simulink model "Eight_Stator_Resistance_Speed_ctrl_of_IM"  (R2024a)
settings: Solver=ode23tb  StartTime=0.0  StopTime=10.0  MaxStep=1e-4  RelTol=1e-3
libraries: spsACVoltageSourceLib x3, spsBreakerLib x3, spsSeriesRLCBranchLib x3, spsAsynchronousMachineSIUnitsLib x1, sps_lib x1
settings Model: Creator=91889  LastModifiedBy=91889
settings DataIOCC: InitialState=[0 0 0 0 0 0 0]  LoadInitialState=on

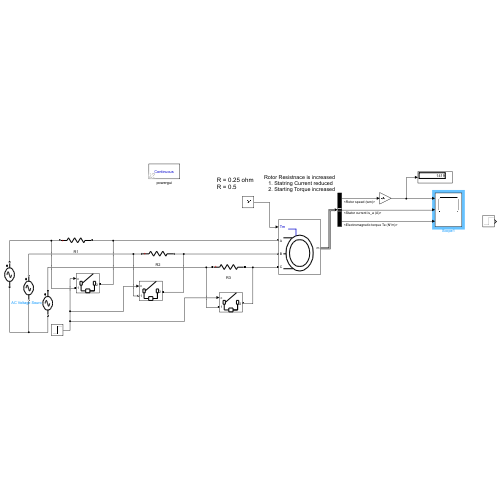
[thumbnail: Simulink's stored preview of the top-level diagram]
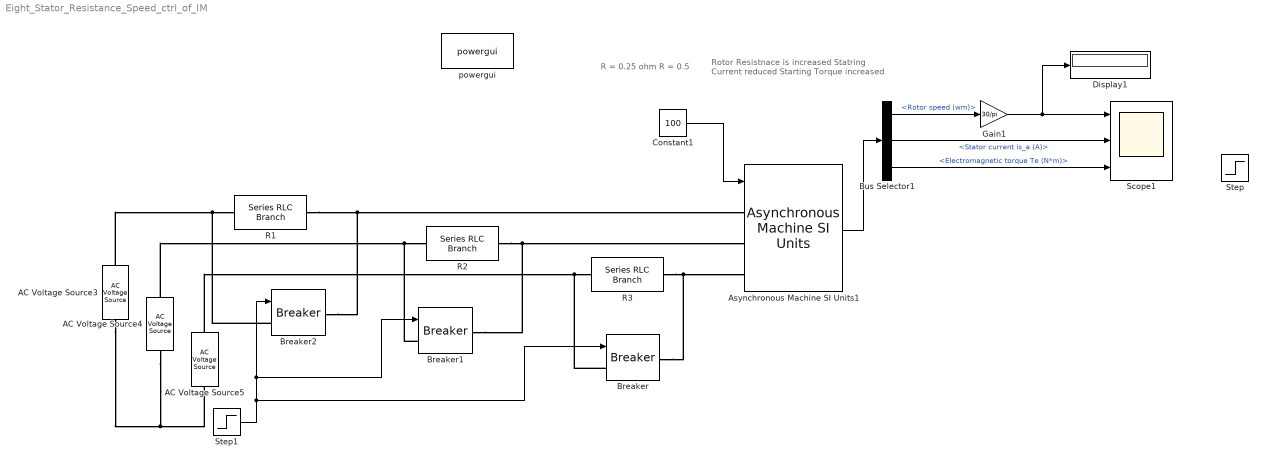
== system Eight_Stator_Resistance_Speed_ctrl_of_IM ==
  note: R = 0.25 ohm
      | R = 0.5
  note: Rotor Resistnace is increased
      | Statring Current reduced
      | Starting Torque increased
  AC Voltage Source3 : spsACVoltageSourceLib/AC Voltage Source  Amplitude=376  Phase=0  Frequency=50  SampleTime=0  Measurements=None  BusType=swing  Pref=10e3  Qref=0  Qmin=-inf  Qmax=+inf
  AC Voltage Source4 : spsACVoltageSourceLib/AC Voltage Source  Amplitude=376  Phase=-120  Frequency=50  SampleTime=0  Measurements=None  BusType=swing  Pref=10e3  Qref=0  Qmin=-inf  Qmax=+inf
  AC Voltage Source5 : spsACVoltageSourceLib/AC Voltage Source  Amplitude=376  Phase=120  Frequency=50  SampleTime=0  Measurements=None  BusType=swing  Pref=10e3  Qref=0  Qmin=-inf  Qmax=+inf
  Asynchronous Machine SI Units1 : spsAsynchronousMachineSIUnitsLib/Asynchronous Machine SI Units  RotorType=Squirrel-cage  PresetModel=No  MechanicalLoad=Torque Tm  ShowDetailedParameters=on  ReferenceFrame=Rotor  Units=SI  MeasurementBus=off  NominalParameters=[1.845e+04 400 50]  VoltageRatio=1  Stator=[0.5968 0.0003495]  Rotor=[0.6258 0.005473]  Cage1=[0.4155 0.002066]  Cage2=[0.4168 0.0003495]  Lm=0.0354  Mechanical=[0.05 0.005879 2]  PolePairs=2  InitialConditions=[0 0 0 0 0 0 0 0]  SimulateSaturation=off  Saturation=[14.03593122, 27.81365428, 53.79336849, 72.68890987, 97.98006896, 148.6815601, 215.7428561, 302.9841135, 428.7778367 ; 230, 322, 414, 460, 506, 552, 598, 644, 690]  LoadFlowParameters=1492000  TsPowergui=0  TsBlock=-1  IterativeModel=Trapezoidal non iterative  IterativeDiscreteModel=Trapezoidal non iterative  Pmec=1.492e+006
  Breaker : spsBreakerLib/Breaker  InitialState=0  SwitchingTimes="[1/60  5/60]"  External=on  BreakerResistance=0.01  SnubberResistance=1e6  SnubberCapacitance=inf  Measurements=None  MoreParameters=on  NoBreakLoop=off
  Breaker1 : spsBreakerLib/Breaker  InitialState=0  SwitchingTimes="[1/60  5/60]"  External=on  BreakerResistance=0.01  SnubberResistance=1e6  SnubberCapacitance=inf  Measurements=None  MoreParameters=on  NoBreakLoop=off
  Breaker2 : spsBreakerLib/Breaker  InitialState=0  SwitchingTimes="[1/60  5/60]"  External=on  BreakerResistance=0.01  SnubberResistance=1e6  SnubberCapacitance=inf  Measurements=None  MoreParameters=on  NoBreakLoop=off
  Bus Selector1 : BusSelector  OutputSignals=Mechanical.Rotor speed (wm),Stator measurements.Stator current is_a (A),Mechanical.Electromagnetic torque Te (N*m)
  Constant1 : Constant  Value=100
  Display1 : Display
  Gain1 : Gain  Gain=30/pi
  R1 : spsSeriesRLCBranchLib/Series RLC Branch  LConnTagsString=__new0  RConnTagsString=__new0  BranchType=R  Resistance=0.01  Inductance=1e-3  SetiL0=off  InitialCurrent=0  Capacitance=1e-6  Setx0=off  InitialVoltage=0  Measurements=None
  R2 : spsSeriesRLCBranchLib/Series RLC Branch  LConnTagsString=__new0  RConnTagsString=__new0  BranchType=R  Resistance=0.01  Inductance=1e-3  SetiL0=off  InitialCurrent=0  Capacitance=1e-6  Setx0=off  InitialVoltage=0  Measurements=None
  R3 : spsSeriesRLCBranchLib/Series RLC Branch  LConnTagsString=__new0  RConnTagsString=__new0  BranchType=R  Resistance=0.01  Inductance=1e-3  SetiL0=off  InitialCurrent=0  Capacitance=1e-6  Setx0=off  InitialVoltage=0  Measurements=None
  Scope1 : Scope  NumInputPorts=3
  Step : Step  Time=0.08  SampleTime=0
  Step1 : Step  Time=0.1  SampleTime=0
  powergui : sps_lib/powergui  Priority=1  SimulationMode=Continuous  SampleTime=50e-6  frequency=60  Iterations=50  frequencyindice=50  Pbase=100e6  ErrMax=1e-4  UnitsV=kV  UnitsW=MW  buscounter=0  FunctionMessages=off  echomessages=off  EnableUseOfTLC=off  CurrentSourceSwitches=off  DisableSnubberDevices=off  DisableRonSwitches=off  DisableVfSwitches=off  DisplayEquations=off  AutomaticDiscreteSolvers=off  SolverType=Tustin/Backward Euler (TBE)  Interpol=off  ExternalGateDelay=off  methode=off  Ts=100  x0status=blocks  SPID=on  SwTol=0  HookPort=off  NonlinearTolerance=1e-4  nMaxIteration=100  ContinueOnMaxIteration=off  RestoreLinks=warning  ResistiveCurrentMeasurement=off  Frange=[0:2:500]  Ylog=off  Xlog=on  ShowGrid=off  save=off  variable=ZData  structure=0  ZoomFFT=off  StartTime=0.0  cycles=1  DisplayStyle=1  fundamental=60  FreqAxis=off  MaxFrequency=1000  frequencyindicesteady=1  RmsSteady=1  display=off
  wires:
  Bus Selector1/1 -> Gain1/1  "<Rotor speed (wm)>"
  Constant1/1 -> Asynchronous Machine SI Units1/1
  Bus Selector1/2 -> Scope1/2  "<Stator current is_a (A)>"
  Bus Selector1/3 -> Scope1/3  "<Electromagnetic torque Te (N*m)>"
  Gain1/1 -> Scope1/1, Display1/1
  Asynchronous Machine SI Units1/1 -> Bus Selector1/1
  Step1/1 -> Breaker/1, Breaker1/1, Breaker2/1
  connections:
  AC Voltage Source4/LConn1 -- AC Voltage Source5/LConn1 -- AC Voltage Source3/LConn1
  AC Voltage Source4/RConn1 -- Breaker1/LConn1 -- R2/LConn1
  AC Voltage Source5/RConn1 -- Breaker/LConn1 -- R3/LConn1
  AC Voltage Source3/RConn1 -- Breaker2/LConn1 -- R1/LConn1
  R1/RConn1 -- Breaker2/RConn1 -- Asynchronous Machine SI Units1/LConn1
  R2/RConn1 -- Breaker1/RConn1 -- Asynchronous Machine SI Units1/LConn2
  R3/RConn1 -- Breaker/RConn1 -- Asynchronous Machine SI Units1/LConn3
